simulink model "Quadrotor_Model_PID_Control_Updated"  (R2023b)
settings: Solver=VariableStepAuto  StartTime=0.0  StopTime=5  MaxStep=1e-2  RelTol=1e-3  AbsTol=1e-3
values from neighbouring files (symbols this model uses):
  b = 1.140 * 10^-7    (= 1.14e-07)    [Quadrotor_PID_Parameter_Trial_Updated.m]
  g = 9.82    [Quadrotor_PID_Parameter_Trial_Updated.m]
  I_xx = 4.856 * 10^-3    (= 0.004856)    [Quadrotor_PID_Parameter_Trial_Updated.m]
  I_yy = 4.856 * 10^-3    (= 0.004856)    [Quadrotor_PID_Parameter_Trial_Updated.m]
  I_zz = 8.801 * 10^-3    (= 0.008801)    [Quadrotor_PID_Parameter_Trial_Updated.m]
  k = 2.980*10^-6    (= 2.98e-06)    [Quadrotor_PID_Parameter_Trial_Updated.m]
  Kdphi = 0.25    [Quadrotor_PID_Parameter_Trial_Updated.m]
  Kdpsi = 0.25    [Quadrotor_PID_Parameter_Trial_Updated.m]
  Kdtheta = 0.25    [Quadrotor_PID_Parameter_Trial_Updated.m]
  Kdx = 0.25    [Quadrotor_PID_Parameter_Trial_Updated.m]
  Kdy = 0.25    [Quadrotor_PID_Parameter_Trial_Updated.m]
  Kdz = 0.25    [Quadrotor_PID_Parameter_Trial_Updated.m]
  Kiphi = 0.25    [Quadrotor_PID_Parameter_Trial_Updated.m]
  Kipsi = 0.25    [Quadrotor_PID_Parameter_Trial_Updated.m]
  Kitheta = 0.25    [Quadrotor_PID_Parameter_Trial_Updated.m]
  Kpphi = 2.5    [Quadrotor_PID_Parameter_Trial_Updated.m]
  Kpphi_attitude = 25    [Quadrotor_PID_Parameter_Trial_Updated.m]
  Kppsi = 2.5    [Quadrotor_PID_Parameter_Trial_Updated.m]
  Kppsi_attitude = 2.5    [Quadrotor_PID_Parameter_Trial_Updated.m]
  Kptheta = 2.5    [Quadrotor_PID_Parameter_Trial_Updated.m]
  Kptheta_attitude = 2.5    [Quadrotor_PID_Parameter_Trial_Updated.m]
  Kzd = 0.25    [Quadrotor_PID_Parameter_Trial_Updated.m]
  Kzi = 0.25    [Quadrotor_PID_Parameter_Trial_Updated.m]
  Kzp = 0.25    [Quadrotor_PID_Parameter_Trial_Updated.m]
  l = 0.225    [Quadrotor_PID_Parameter_Trial_Updated.m]    (also in Reference_Drone_Updated_PID.m = 0.15)
  m = 0.468    [Quadrotor_PID_Parameter_Trial_Updated.m]
  pitch_d = 0.01    [Quadrotor_PID_Parameter_Trial_Updated.m]
  roll_d = 0.01    [Quadrotor_PID_Parameter_Trial_Updated.m]
  yaw_d = 0.01    [Quadrotor_PID_Parameter_Trial_Updated.m]
  z_d = 1    [Quadrotor_PID_Parameter_Trial_Updated.m]
settings Model: Creator=jerss  LastModifiedBy=jerss

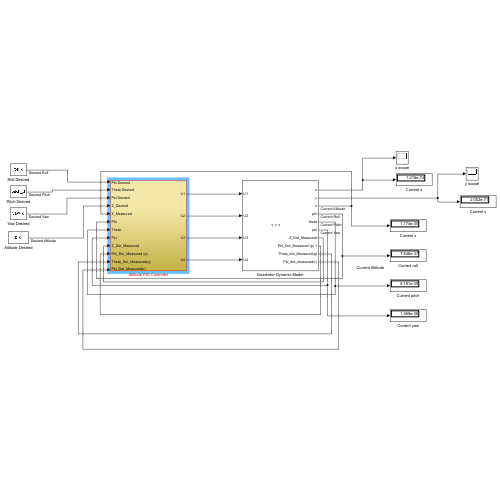
[thumbnail: Simulink's stored preview of the top-level diagram]
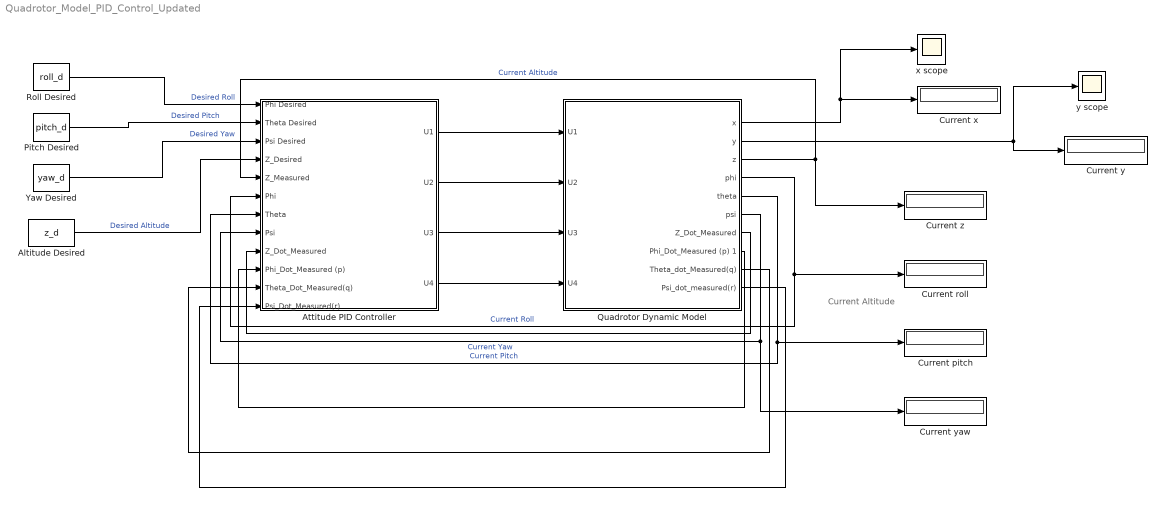
== system Quadrotor_Model_PID_Control_Updated ==
  note: Current Altitude
  Altitude Desired : Constant  Value=z_d
  Attitude PID Controller : Subsystem
  Current pitch : Display
  Current roll : Display
  Current x : Display
  Current y : Display
  Current yaw : Display
  Current z : Display
  Pitch Desired : Constant  Value=pitch_d
  Quadrotor Dynamic Model : Subsystem
      mask Display: image('C:\Users\angel\OneDrive - Universidad Politécnica de Yucatán\CIMAT\1st semester\Robotic Systems Modeling and Control\Project\Quadrotor\images\quadrotor.jpg');
  Roll Desired : Constant  Value=roll_d
  Yaw Desired : Constant  Value=yaw_d
  x scope : Scope
  y scope : Scope
  wires:
  Quadrotor Dynamic Model/3(z) -> Current z/1, Attitude PID Controller/5(Z_Measured)  "Current Altitude"
  Quadrotor Dynamic Model/4(phi) -> Current roll/1, Attitude PID Controller/6(Phi)  "Current Roll"
  Quadrotor Dynamic Model/5(theta) -> Current pitch/1, Attitude PID Controller/7(Theta)  "Current Pitch"
  Quadrotor Dynamic Model/6(psi) -> Current yaw/1, Attitude PID Controller/8(Psi)  "Current Yaw"
  Attitude PID Controller/1(U1) -> Quadrotor Dynamic Model/1(U1)
  Attitude PID Controller/2(U2) -> Quadrotor Dynamic Model/2(U2)
  Attitude PID Controller/3(U3) -> Quadrotor Dynamic Model/3(U3)
  Attitude PID Controller/4(U4) -> Quadrotor Dynamic Model/4(U4)
  Roll Desired/1 -> Attitude PID Controller/1(Phi Desired)  "Desired Roll"
  Pitch Desired/1 -> Attitude PID Controller/2(Theta Desired)  "Desired Pitch"
  Yaw Desired/1 -> Attitude PID Controller/3(Psi Desired)  "Desired Yaw"
  Altitude Desired/1 -> Attitude PID Controller/4(Z_Desired)  "Desired Altitude"
  Quadrotor Dynamic Model/1(x) -> x scope/1, Current x/1
  Quadrotor Dynamic Model/2(y) -> y scope/1, Current y/1
  Quadrotor Dynamic Model/7(Z_Dot_Measured) -> Attitude PID Controller/9(Z_Dot_Measured)
  Quadrotor Dynamic Model/8(Phi_Dot_Measured (p) 1) -> Attitude PID Controller/10(Phi_Dot_Measured (p))
  Quadrotor Dynamic Model/9(Theta_dot_Measured(q)) -> Attitude PID Controller/11(Theta_Dot_Measured(q))
  Quadrotor Dynamic Model/10(Psi_dot_measured(r)) -> Attitude PID Controller/12(Psi_Dot_Measured(r))

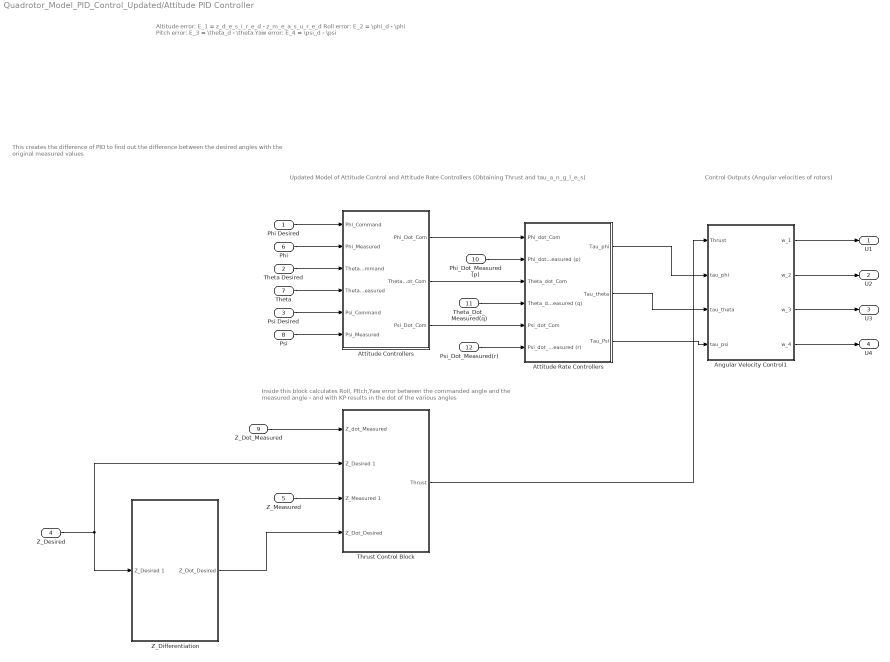
== system Quadrotor_Model_PID_Control_Updated/Attitude PID Controller ==
  note: Inside this block calculates Roll, PItch,Yaw error between the commanded angle and the measured angle - and with KP results in the dot of the various angles
  note: This creates the difference of PID to find out the difference between the desired angles with the original measured values
  note: Altitude error: E_1 = z_d_e_s_i_r_e_d - z_m_e_a_s_u_r_e_d
      | Roll error: E_2 = \phi_d - \phi
      | Pitch error: E_3 = \theta_d - \theta
      | Yaw error: E_4 = \psi_d - \psi
  note: Updated Model of Attitude Control and Attitude Rate Controllers
      | (Obtaining Thrust and tau_a_n_g_l_e_s)
  note: Control Outputs
      | (Angular velocities of rotors)
  Phi Desired : Inport
  Theta Desired : Inport  Port=2
  Psi Desired : Inport  Port=3
  Z_Desired : Inport  Port=4
  Z_Measured : Inport  Port=5
  Phi : Inport  Port=6
  Theta : Inport  Port=7
  Psi : Inport  Port=8
  Z_Dot_Measured : Inport  Port=9
  Phi_Dot_Measured (p) : Inport  Port=10
  Theta_Dot_Measured(q) : Inport  Port=11
  Psi_Dot_Measured(r) : Inport  Port=12
  Angular Velocity Control1 : Subsystem
  Attitude Controllers : Subsystem
  "Attitude Rate Controllers " : Subsystem
  Thrust Control Block : Subsystem
  Z_Differentiation : Subsystem
  U1 : Outport
  U2 : Outport  Port=2
  U3 : Outport  Port=3
  U4 : Outport  Port=4
  wires:
  Attitude Controllers/1(Phi_Dot_Com) -> "Attitude Rate Controllers "/1(Phi_dot_Com)
  Attitude Controllers/2(Theta_Dot_Com) -> "Attitude Rate Controllers "/3(Theta_dot_Com)
  Attitude Controllers/3(Psi_Dot_Com) -> "Attitude Rate Controllers "/5("Psi_dot_Com ")
  Angular Velocity Control1/4("w_4 ") -> U4/1
  Angular Velocity Control1/3(w_3) -> U3/1
  Angular Velocity Control1/2(w_2) -> U2/1
  Angular Velocity Control1/1(w_1) -> U1/1
  Thrust Control Block/1(Thrust) -> Angular Velocity Control1/1(Thrust)
  "Attitude Rate Controllers "/1(Tau_phi) -> Angular Velocity Control1/2(tau_phi)
  "Attitude Rate Controllers "/2(Tau_theta) -> Angular Velocity Control1/3(tau_theta)
  "Attitude Rate Controllers "/3(Tau_Psi) -> Angular Velocity Control1/4("tau_psi ")
  Z_Differentiation/1(Z_Dot_Desired) -> Thrust Control Block/4(Z_Dot_Desired)
  Phi Desired/1 -> Attitude Controllers/1(Phi_Command)
  Psi Desired/1 -> Attitude Controllers/5("Psi_Command ")
  Theta Desired/1 -> Attitude Controllers/3(Theta_Command)
  Phi/1 -> Attitude Controllers/2(Phi_Measured)
  Z_Desired/1 -> Thrust Control Block/2(Z_Desired 1), Z_Differentiation/1(Z_Desired 1)
  Z_Measured/1 -> Thrust Control Block/3(Z_Measured 1)
  Psi/1 -> Attitude Controllers/6("Psi_Measured ")
  Theta/1 -> Attitude Controllers/4(Theta_Measured)
  Z_Dot_Measured/1 -> Thrust Control Block/1(Z_dot_Measured)
  Phi_Dot_Measured (p)/1 -> "Attitude Rate Controllers "/2(Phi_dot_Measured (p))
  Theta_Dot_Measured(q)/1 -> "Attitude Rate Controllers "/4(Theta_dot_Measured (q))
  Psi_Dot_Measured(r)/1 -> "Attitude Rate Controllers "/6("Psi_dot_Measured (r) ")

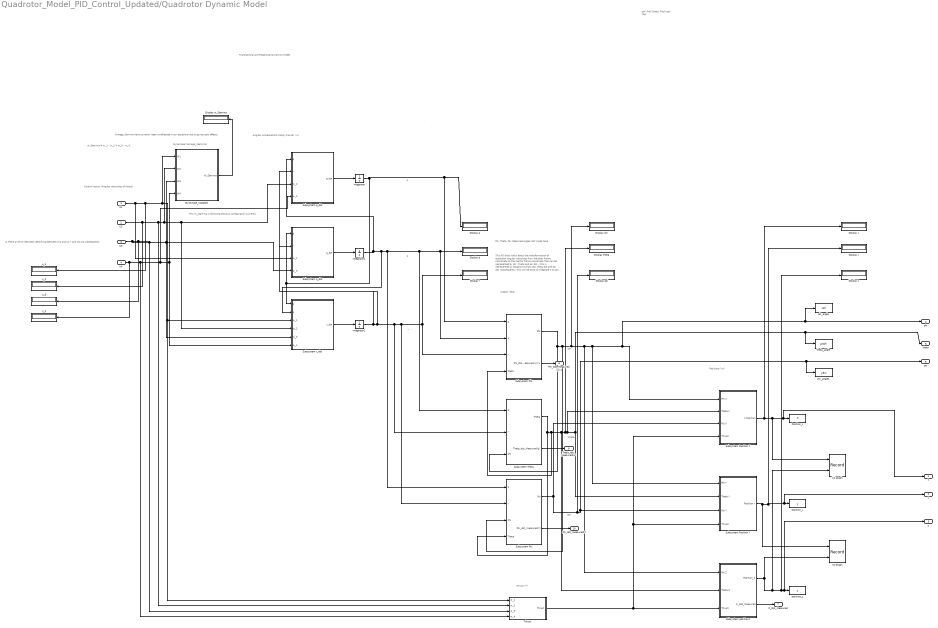
== system Quadrotor_Model_PID_Control_Updated/Quadrotor Dynamic Model ==
  note: w_Gamma = w_1 - w_2 + w_3 - w_4;
  note: Is there an error between identifying between W1 and U1 ? and W2,U2 subsequently
  note: Phi, Theta, Psi Measured angles dot inside here
  note: This W_Gamma is following the plus configuration currently
  note: Omega_Gamma have currently been unreflected in our equations due to gyroscopic effects
  note: This full block talks about the trabsformation of quadrotor angular velocities from the body frame coordinate to the inertial frame coordinate that can be represented by phi , theta and psi dot - this is represented by equation 6 of phi dot, theta dot and psi dot.
      | Subsequently, this will be done to integrate it to phi, theta and psi.
  note: Angular Accelerations (Body Frame) (\nu)
  note: .
  note: \phi: Roll
      | \theta: Pitch
      | \psi: Yaw
  note: Control Inputs
      | (Angular velocities of rotors)
  note: Positions (\xi)
  note: Angles (\eta)
  note: Gyroscope (\omega_\Gamma)
  note: Thrust (T)
  note: p
  note: q
  note: r
  note: \phi
  note: \theta
  note: \psi
  note: Translational and Rotational Dynamics Model
  U1 : Inport
  U2 : Inport  Port=2
  U3 : Inport  Port=3
  U4 : Inport  Port=4
  Display p : Display
  Display phi : Display
  Display psi : Display
  Display q : Display
  Display r : Display
  Display theta : Display
  Display w_Gamma : Display
  Display x : Display
  Display y : Display
  Display z : Display
  Gyroscope_Updated : Subsystem
  Integrator : Integrator
  Integrator1 : Integrator
  Integrator2 : Integrator
  Position_x : ToWorkspace  VariableName=X  SampleTime=-1
  Subsystem Phi : Subsystem
  Subsystem Position X : Subsystem
  Subsystem Position Y : Subsystem
  Subsystem Psi : Subsystem
  Subsystem Theta : Subsystem
  Subsystem p_dot : Subsystem
  Subsystem position z : Subsystem
  Subsystem q_dot : Subsystem
  Subsystem r_dot : Subsystem
  Thrust : MATLAB Function  TreatAsAtomicUnit=on
  XZ graph : Record  FileSettingsInternal="{\"entries\":[{\"content\":{\"excelSettings\":{\"content\":{},\"type\":\"Streamout.ExcelSettings\"}},\"type\":\"Streamout.FileSettingStorage\",\"uuid\":\"\"}],\"packageUris\":[\"http:\\/\\/schema.mathworks.com\\/mf0\\/streamout_blocks\\/R2020a\"],\"version\":\"1.0\"}"  Layout=[1 1]  SignalsInternal="{\"entries\":[{\"content\":{\"signals\":[{\"content\":{\"blockPath\":[],\"dimensions\":[1],\"domain\":\"\",\"lineColor\":\"#a2142f\",\"plots\":[1],\"port\":1,\"sid\":[\"\"],\"signalID\":59066,\"signalName\":\"Subsystem Position X\"},\"type\":\"RecordBlkView.Signal\",\"uuid\":\"\"},{\"content\":{\"blockPath\":[],\"dimensions\":[1],\"domain\":\"\",\"lineColor\":\"#139fff\",\"plots\":[1],\"port\":2,\"sid\":[\"\"],\"signalID\":59070,\"signalName\":\"Subsystem position z:1\"},\"type\":\"RecordBlkView.Signal\",\"uuid\":\"\"}]},\"type\":\"RecordBlkView.InputSignals\",\"uuid\":\"\"}],\"packageUris\":[\"http:\\/\\/schema.mathworks.com\\/mf0\\/streamout_blocks\\/R2020a\"],\"version\":\"1.0\"}"  VisualizationBindings="{\"xyplotplugin\":{\"info\":[{\"series\":[{\"bindingParametersList\":[{\"parameter\":\"X-Axis\",\"signalID\":59066,\"signalName\":\"Subsystem Position X\"},{\"parameter\":\"Y-Axis\",\"signalID\":59070,\"signalName\":\"Subsystem position z:1\"}],\"seriesID\":430}],\"subplotID\":1}]}}"  CompatibilityTag=XY  st=-1
  YZ Graph : Record  FileSettingsInternal="{\"entries\":[{\"content\":{\"excelSettings\":{\"content\":{},\"type\":\"Streamout.ExcelSettings\"}},\"type\":\"Streamout.FileSettingStorage\",\"uuid\":\"\"}],\"packageUris\":[\"http:\\/\\/schema.mathworks.com\\/mf0\\/streamout_blocks\\/R2020a\"],\"version\":\"1.0\"}"  Layout=[1 1]  SignalsInternal="{\"entries\":[{\"content\":{\"signals\":[{\"content\":{\"blockPath\":[],\"dimensions\":[1],\"domain\":\"\",\"lineColor\":\"#a2142f\",\"plots\":[1],\"port\":1,\"sid\":[\"\"],\"signalID\":59074,\"signalName\":\"Subsystem Position Y\"},\"type\":\"RecordBlkView.Signal\",\"uuid\":\"\"},{\"content\":{\"blockPath\":[],\"dimensions\":[1],\"domain\":\"\",\"lineColor\":\"#139fff\",\"plots\":[1],\"port\":2,\"sid\":[\"\"],\"signalID\":59078,\"signalName\":\"Subsystem position z:1\"},\"type\":\"RecordBlkView.Signal\",\"uuid\":\"\"}]},\"type\":\"RecordBlkView.InputSignals\",\"uuid\":\"\"}],\"packageUris\":[\"http:\\/\\/schema.mathworks.com\\/mf0\\/streamout_blocks\\/R2020a\"],\"version\":\"1.0\"}"  VisualizationBindings="{\"xyplotplugin\":{\"info\":[{\"series\":[{\"bindingParametersList\":[{\"parameter\":\"X-Axis\",\"signalID\":59074,\"signalName\":\"Subsystem Position Y\"},{\"parameter\":\"Y-Axis\",\"signalID\":59078,\"signalName\":\"Subsystem position z:1\"}],\"seriesID\":13612}],\"subplotID\":1}]}}"  CompatibilityTag=XY  st=-1
  phi_angle : ToWorkspace  VariableName=roll  SampleTime=-1
  phi_angle1 : ToWorkspace  VariableName=yaw  SampleTime=-1
  position_y : ToWorkspace  VariableName=y  SampleTime=-1
  position_z : ToWorkspace  VariableName=z  SampleTime=-1
  theta_angle : ToWorkspace  VariableName=pitch  SampleTime=-1
  u_{1..4} (4 alike) : Display
  x : Outport
  y : Outport  Port=2
  z : Outport  Port=3
  phi : Outport  Port=4
  theta : Outport  Port=5
  psi : Outport  Port=6
  Z_Dot_Measured : Outport  Port=7
  Phi_Dot_Measured (p) 1 : Outport  Port=8
  Theta_dot_Measured(q) : Outport  Port=9
  Psi_dot_measured(r) : Outport  Port=10
  wires:
  U1/1 -> Subsystem q_dot/3(w_1), u_1/1, Gyroscope_Updated/1(W1), Subsystem r_dot/3(w_1), Thrust/1(w_1)
  U2/1 -> Gyroscope_Updated/2(W2), Subsystem p_dot/3(w_2), Subsystem r_dot/4(w_2), Thrust/2(w_2), u_2/1
  U3/1 -> Subsystem q_dot/4(w_3), Gyroscope_Updated/3(W3), Subsystem r_dot/5(w_3), Thrust/3(w_3), u_3/1
  U4/1 -> u_4/1, Gyroscope_Updated/4(W4), Subsystem r_dot/6(w_4), Subsystem p_dot/4(w_4), Thrust/4(w_4)
  Thrust/1(Thrust) -> Subsystem Position X/4(Thrust), Subsystem Position Y/4("Thrust "), Subsystem position z/3(Thrust)
  Subsystem Phi/1("Phi ") -> Subsystem Theta/3("phi "), Subsystem Psi/3(Phi), Display phi/1, Subsystem position z/1("Phi Z "), Subsystem Position Y/1("Phi Y "), phi/1, phi_angle/1, Subsystem Position X/1("Phi X ")
  Subsystem Psi/1(Psi) -> Display psi/1, phi_angle1/1, psi/1, Subsystem Position Y/3("Psi Y "), Subsystem Position X/3("Psi X ")
  Subsystem Position X/1(X Position) -> Display x/1, x/1, Position_x/1, XZ graph/1
  Subsystem position z/1(Position_Z) -> XZ graph/2, z/1, position_z/1, Display z/1, YZ Graph/2
  Subsystem Position Y/1("Position Y ") -> y/1, position_y/1, Display y/1, YZ Graph/1
  Gyroscope_Updated/1(W_Gamma) -> Display w_Gamma/1
  Subsystem p_dot/1(p_dot) -> Integrator/1
  Subsystem q_dot/1(q_dot) -> Integrator1/1
  Subsystem r_dot/1(r_dot) -> Integrator2/1
  Integrator/1 -> Display p/1, Subsystem Phi/1(p), Subsystem r_dot/1("p "), Subsystem q_dot/1("p ")
  Integrator2/1 -> Subsystem Theta/2(r), Subsystem Psi/2(r), Display r/1, Subsystem Phi/3(r), Subsystem p_dot/2(r), Subsystem q_dot/2(r)
  Integrator1/1 -> Subsystem p_dot/1(q), Subsystem Psi/1(q), Subsystem Theta/1(q), Display q/1, Subsystem Phi/2(q), Subsystem r_dot/2(q)
  Subsystem Theta/1(Theta) -> Subsystem Psi/4(Theta), Subsystem Phi/4(theta), Subsystem position z/2("Theta Z "), Display theta/1, Subsystem Position X/2("Theta X "), theta_angle/1, theta/1, Subsystem Position Y/2("Theta Y ")
  Subsystem position z/2(Z_Dot_Measured) -> Z_Dot_Measured/1
  Subsystem Phi/2(Phi_Dot_Measured (p) 1) -> Phi_Dot_Measured (p) 1/1
  Subsystem Theta/2(Theta_dot_Measured(q)) -> Theta_dot_Measured(q)/1
  Subsystem Psi/2(Psi_dot_measured(r)) -> Psi_dot_measured(r)/1

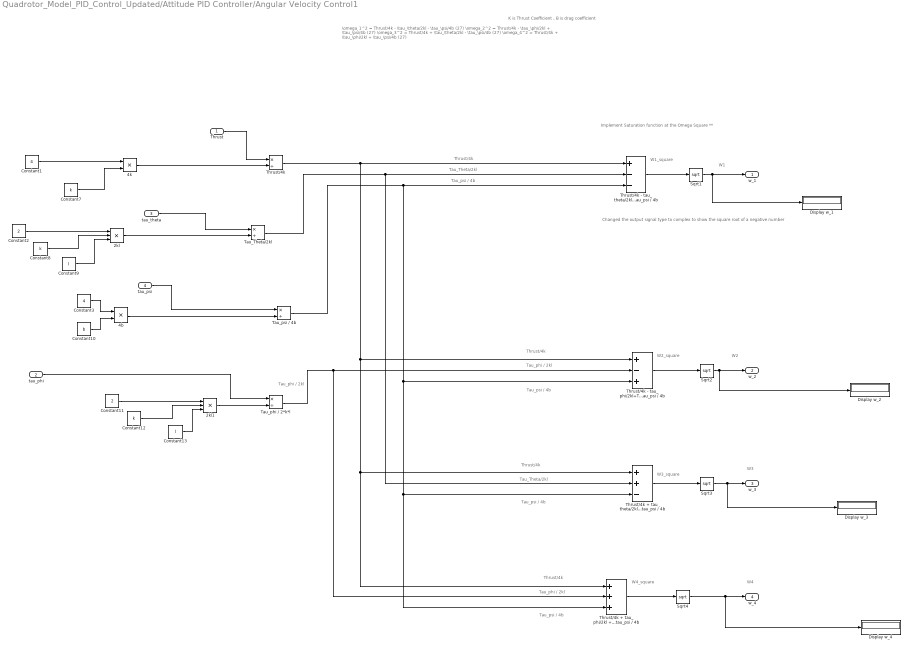
== system Quadrotor_Model_PID_Control_Updated/Attitude PID Controller/Angular Velocity Control1 ==
  note: Implement Saturation function at the Omega Square **
  note: Changed the output signal type to complex to show the square root of a negative number
  note: Tau_psi / 4b
  note: Tau_Theta/2kl
  note: Thrust/4k
  note: W1_square
  note: K is Thrust Coefficient , B is drag coefficient
  note: \omega_1^2 = Thrust/4k - \tau_\theta/2kl - \tau_\psi/4b   (27)
      |
      | \omega_2^2 = Thrust/4k - \tau_\phi/2kl + \tau_\psi/4b   (27)
      |
      | \omega_3^2 = Thrust/4k + \tau_\theta/2kl - \tau_\psi/4b   (27)
      |
      | \omega_4^2 = Thrust/4k + \tau_\phi/2kl + \tau_\psi/4b   (27)
  note: W1
  note: Thrust/4k
  note: Tau_phi / 2kl
  note: Tau_psi / 4b
  note: W2_square
  note: W2
  note: Thrust/4k
  note: W3
  note: W3_square
  note: Tau_Theta/2kl
  note: Tau_psi / 4b
  note: W4_square
  note: W4
  note: Thrust/4k
  note: Tau_phi / 2kl
  note: Tau_phi / 2kl
  note: Tau_psi / 4b
  Thrust : Inport
  tau_phi : Inport  Port=2
  tau_theta : Inport  Port=3
  "tau_psi " : Inport  Port=4
  2kl : Product  Inputs=***
  2kl1 : Product  Inputs=***
  4b : Product  Inputs=**
  4k : Product  Inputs=**
  Constant1 : Constant  Value=4
  Constant10 : Constant  Value=b
  Constant11 : Constant  Value=2
  Constant12 : Constant  Value=k
  Constant13 : Constant  Value=l
  Constant2 : Constant  Value=2
  Constant3 : Constant  Value=4
  Constant7 : Constant  Value=k
  Constant8 : Constant  Value=k
  Constant9 : Constant  Value=l
  Display w_{1..4} (4 alike) : Display
  Sqrt1 : Sqrt
  Sqrt2 : Sqrt  OutputSignalType=real
  Sqrt3 : Sqrt
  Sqrt4 : Sqrt
  Tau_Theta/2kl : Product  Inputs=*/
  Tau_phi / 2*k*l : Product  Inputs=*/
  Tau_psi / 4b : Product  Inputs=*/
  Thrust/4k : Product  Inputs=*/
  Thrust/4k + tau_phi/2kl + tau_psi / 4b : Sum  Inputs=+++
  Thrust/4k + tau_theta/2kl -tau_psi / 4b : Sum  Inputs=++-
  Thrust/4k - tau_phi/2kl+Tau_psi / 4b : Sum  Inputs=+-+
  Thrust/4k - tau_theta/2kl-Tau_psi / 4b : Sum  Inputs=+--
  w_1 : Outport
  w_2 : Outport  Port=2
  w_3 : Outport  Port=3
  "w_4 " : Outport  Port=4
  wires:
  tau_theta/1 -> Tau_Theta/2kl/1
  Sqrt1/1 -> Display w_1/1, w_1/1
  tau_phi/1 -> Tau_phi / 2*k*l/1
  "tau_psi "/1 -> Tau_psi / 4b/1
  Sqrt2/1 -> Display w_2/1, w_2/1
  Thrust/4k - tau_phi/2kl+Tau_psi / 4b/1 -> Sqrt2/1
  Thrust/4k + tau_theta/2kl -tau_psi / 4b/1 -> Sqrt3/1
  Sqrt3/1 -> Display w_3/1, w_3/1
  Thrust/4k + tau_phi/2kl + tau_psi / 4b/1 -> Sqrt4/1
  Sqrt4/1 -> Display w_4/1, "w_4 "/1
  Constant1/1 -> 4k/1
  Constant7/1 -> 4k/2
  Constant8/1 -> 2kl/2
  Constant2/1 -> 2kl/1
  2kl/1 -> Tau_Theta/2kl/2
  Constant9/1 -> 2kl/3
  Constant3/1 -> 4b/1
  Constant10/1 -> 4b/2
  4k/1 -> Thrust/4k/2
  Constant11/1 -> 2kl1/1
  Constant12/1 -> 2kl1/2
  Constant13/1 -> 2kl1/3
  Thrust/1 -> Thrust/4k/1
  4b/1 -> Tau_psi / 4b/2
  2kl1/1 -> Tau_phi / 2*k*l/2
  Thrust/4k/1 -> Thrust/4k + tau_theta/2kl -tau_psi / 4b/1, Thrust/4k + tau_phi/2kl + tau_psi / 4b/1, Thrust/4k - tau_phi/2kl+Tau_psi / 4b/1, Thrust/4k - tau_theta/2kl-Tau_psi / 4b/1
  Tau_Theta/2kl/1 -> Thrust/4k - tau_theta/2kl-Tau_psi / 4b/2, Thrust/4k + tau_theta/2kl -tau_psi / 4b/2
  Thrust/4k - tau_theta/2kl-Tau_psi / 4b/1 -> Sqrt1/1
  Tau_phi / 2*k*l/1 -> Thrust/4k + tau_phi/2kl + tau_psi / 4b/2, Thrust/4k - tau_phi/2kl+Tau_psi / 4b/2
  Tau_psi / 4b/1 -> Thrust/4k - tau_theta/2kl-Tau_psi / 4b/3, Thrust/4k - tau_phi/2kl+Tau_psi / 4b/3, Thrust/4k + tau_phi/2kl + tau_psi / 4b/3, Thrust/4k + tau_theta/2kl -tau_psi / 4b/3

== system Quadrotor_Model_PID_Control_Updated/Attitude PID Controller/Attitude Controllers ==
  note: Phi,Theta, Psi dot measured can be taken from the UAV Quadrotor Modelling
  note: Taken from Iris + Quadrotor Equations - on Attitude Controllers - Equation 57,58,59 - Can also follow 49.50.51.52.53 Eqn
  note: Yaw Rate Command
  note: Pitch Rate Command
  note: Roll Rate Command
  note: Utilising PD to minimise error in Z-Axis
      | Total Thrust T which affects the acceleration in the z- direction is set to equal to mg.
      | Constraint is enforced to keep the quadcopter flying.
      | Converting thrust equation to appropriate reference frame and utisiling PD to minimise the error in the Z-Axis
      |
      | T = (g + K_{z,D}(z_d_e_s_i_r_e_ddot - z_d_o_t) + K_{z,P}(z_d_e_s_i_r_e_d - z)) m/(C_\phiC_\theta)     (25)
      |
      | \tau_\phi = (K_{\phi,D}(\phi_d - \phi) + K_{\phi,P}(\phi_d - \phi)) I_{xx}                   (24)
      |
      | \tau_\theta = (K_{\theta,D}(\theta_d - \theta) + K_{\theta,P}(\theta_d - \theta)) I_{yy}                    (24)
      |
      | \tau_\psi = (K_{\psi,D}(\psi_d - \psi) + K_{\psi,P}(\psi_d - \psi)) I_{zz}                (24)
  Phi_Command : Inport
  Phi_Measured : Inport  Port=2
  Theta_Command : Inport  Port=3
  Theta_Measured : Inport  Port=4
  "Psi_Command " : Inport  Port=5
  "Psi_Measured " : Inport  Port=6
  Pitch error : Display
  Proportional Gain : Gain  Gain=Kpphi_attitude
  Proportional Gain1 : Gain  Gain=Kptheta_attitude
  Proportional Gain2 : Gain  Gain=Kppsi_attitude
  Roll error : Display
  Sum1 : Sum  Inputs=|+-
  Sum2 : Sum  Inputs=|+-
  Sum3 : Sum  Inputs=|+-
  Yaw error : Display
  Phi_Dot_Com : Outport
  Theta_Dot_Com : Outport  Port=2
  Psi_Dot_Com : Outport  Port=3
  wires:
  Phi_Command/1 -> Sum3/1
  Phi_Measured/1 -> Sum3/2
  Sum3/1 -> Roll error/1, Proportional Gain/1  "Roll Error"
  Theta_Command/1 -> Sum2/1
  Theta_Measured/1 -> Sum2/2
  Sum2/1 -> Pitch error/1, Proportional Gain1/1  "Pitch Error"
  "Psi_Command "/1 -> Sum1/1
  "Psi_Measured "/1 -> Sum1/2
  Sum1/1 -> Yaw error/1, Proportional Gain2/1  "Yaw Error"
  Proportional Gain/1 -> Phi_Dot_Com/1
  Proportional Gain1/1 -> Theta_Dot_Com/1
  Proportional Gain2/1 -> Psi_Dot_Com/1

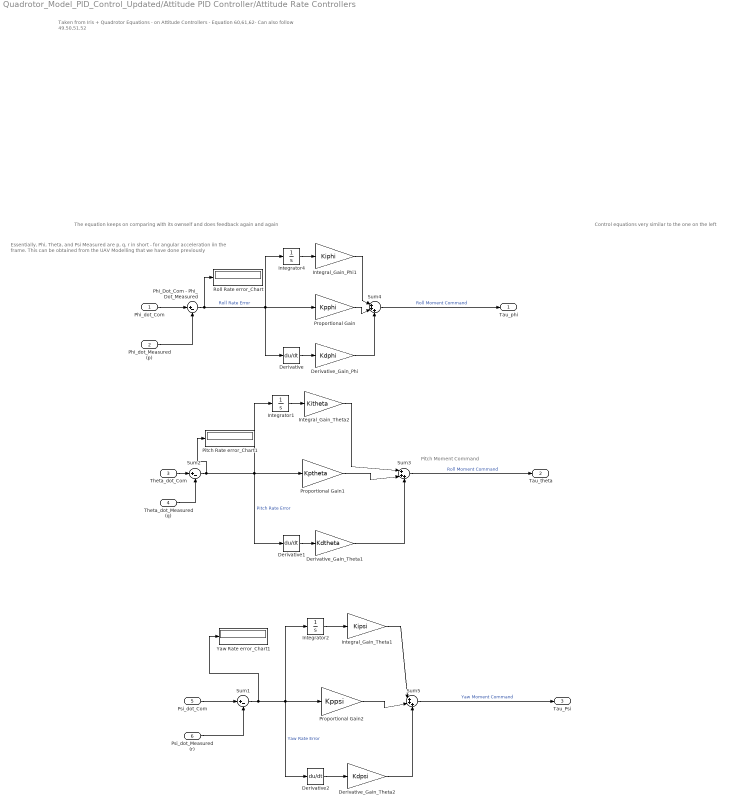
== system Quadrotor_Model_PID_Control_Updated/Attitude PID Controller/Attitude Rate Controllers  ==
  note: Essentially, Phi, Theta, and Psi Measured are p, q, r in short - for angular acceleration iin the frame. This can be obtained from the UAV Modelling that we have done previously
  note: Control equations very similar to the one on the left
  note: The equation keeps on comparing with its ownself and does feedback again and again
  note: Taken from Iris + Quadrotor Equations - on Attitude Controllers - Equation 60,61,62- Can also follow 49.50,51.52
  note: Pitch Moment Command
  Phi_dot_Com : Inport
  Phi_dot_Measured (p) : Inport  Port=2
  Theta_dot_Com : Inport  Port=3
  Theta_dot_Measured (q) : Inport  Port=4
  "Psi_dot_Com " : Inport  Port=5
  "Psi_dot_Measured (r) " : Inport  Port=6
  Derivative : Derivative
  Derivative1 : Derivative
  Derivative2 : Derivative
  Derivative_Gain_Phi : Gain  Gain=Kdphi
  Derivative_Gain_Theta1 : Gain  Gain=Kdtheta
  Derivative_Gain_Theta2 : Gain  Gain=Kdpsi
  Integral_Gain_Phi1 : Gain  Gain=Kiphi
  Integral_Gain_Theta1 : Gain  Gain=Kipsi
  Integral_Gain_Theta2 : Gain  Gain=Kitheta
  Integrator1 : Integrator
  Integrator2 : Integrator
  Integrator4 : Integrator
  Phi_Dot_Com - Phi_Dot_Measured : Sum  Inputs=|+-
  Pitch Rate error_Chart1 : Display
  Proportional Gain : Gain  Gain=Kpphi
  Proportional Gain1 : Gain  Gain=Kptheta
  Proportional Gain2 : Gain  Gain=Kppsi
  Roll Rate error_Chart : Display
  Sum1 : Sum  Inputs=|+-
  Sum2 : Sum  Inputs=|+-
  Sum3 : Sum  Inputs=|+++
  Sum4 : Sum  Inputs=|+++
  Sum5 : Sum  Inputs=|+++
  Yaw Rate error_Chart1 : Display
  Tau_phi : Outport
  Tau_theta : Outport  Port=2
  Tau_Psi : Outport  Port=3
  wires:
  Phi_dot_Com/1 -> Phi_Dot_Com - Phi_Dot_Measured/1
  Phi_dot_Measured (p)/1 -> Phi_Dot_Com - Phi_Dot_Measured/2
  Phi_Dot_Com - Phi_Dot_Measured/1 -> Roll Rate error_Chart/1, Integrator4/1, Derivative/1, Proportional Gain/1  "Roll Rate Error"
  Theta_dot_Com/1 -> Sum2/1
  Theta_dot_Measured (q)/1 -> Sum2/2
  Sum2/1 -> Pitch Rate error_Chart1/1, Derivative1/1, Integrator1/1, Proportional Gain1/1  "Pitch Rate Error"
  "Psi_dot_Com "/1 -> Sum1/1
  "Psi_dot_Measured (r) "/1 -> Sum1/2
  Sum1/1 -> Yaw Rate error_Chart1/1, Derivative2/1, Integrator2/1, Proportional Gain2/1  "Yaw Rate Error"
  Sum4/1 -> Tau_phi/1  "Roll Moment Command"
  Derivative/1 -> Derivative_Gain_Phi/1
  Integral_Gain_Phi1/1 -> Sum4/1
  Proportional Gain/1 -> Sum4/2
  Derivative_Gain_Phi/1 -> Sum4/3
  Integrator4/1 -> Integral_Gain_Phi1/1
  Integral_Gain_Theta2/1 -> Sum3/1
  Integrator1/1 -> Integral_Gain_Theta2/1
  Proportional Gain1/1 -> Sum3/2
  Derivative1/1 -> Derivative_Gain_Theta1/1
  Derivative_Gain_Theta1/1 -> Sum3/3
  Sum3/1 -> Tau_theta/1  "Roll Moment Command"
  Integral_Gain_Theta1/1 -> Sum5/1
  Integrator2/1 -> Integral_Gain_Theta1/1
  Sum5/1 -> Tau_Psi/1  "Yaw Moment Command"
  Proportional Gain2/1 -> Sum5/2
  Derivative2/1 -> Derivative_Gain_Theta2/1
  Derivative_Gain_Theta2/1 -> Sum5/3

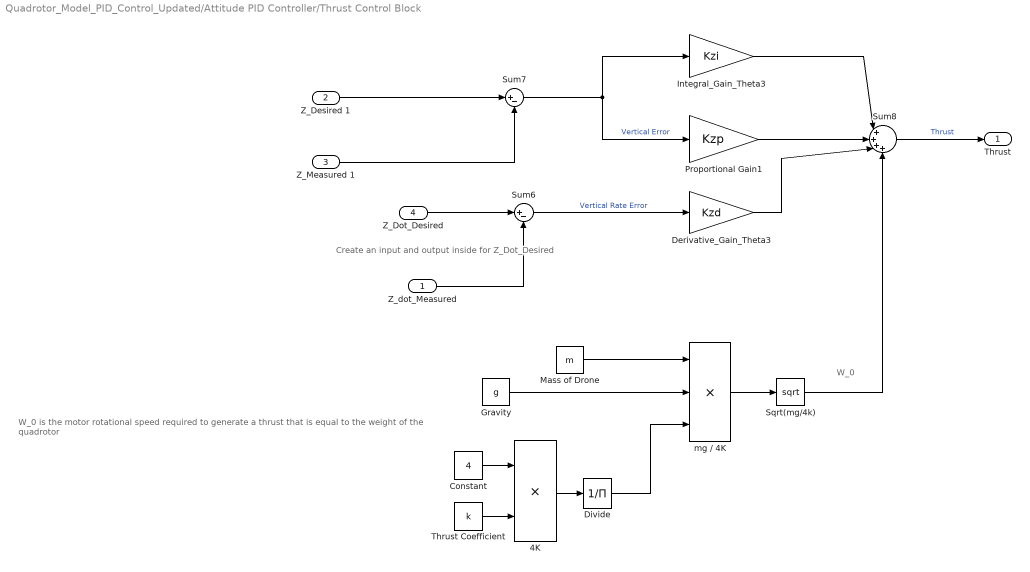
== system Quadrotor_Model_PID_Control_Updated/Attitude PID Controller/Thrust Control Block ==
  note: Create an input and output inside for Z_Dot_Desired
  note: W_0
  note: W_0 is the motor rotational speed required to generate a thrust that is equal to the weight of the quadrotor
  Z_dot_Measured : Inport
  Z_Desired 1 : Inport  Port=2
  Z_Measured 1 : Inport  Port=3
  Z_Dot_Desired : Inport  Port=4
  4K : Product
  Constant : Constant  Value=4
  Derivative_Gain_Theta3 : Gain  Gain=Kzd
  Divide : Product  Inputs=/
  Gravity : Constant  Value=g
  Integral_Gain_Theta3 : Gain  Gain=Kzi
  Mass of Drone : Constant  Value=m
  Proportional Gain1 : Gain  Gain=Kzp
  Sqrt(mg/4k) : Sqrt
  Sum6 : Sum  Inputs=|+-
  Sum7 : Sum  Inputs=|+-
  Sum8 : Sum  Inputs=|++++
  Thrust Coefficient : Constant  Value=k
  mg / 4K : Product  Inputs=3
  Thrust : Outport
  wires:
  Sqrt(mg/4k)/1 -> Sum8/4
  Sum8/1 -> Thrust/1  "Thrust"
  Integral_Gain_Theta3/1 -> Sum8/1
  Z_dot_Measured/1 -> Sum6/2
  mg / 4K/1 -> Sqrt(mg/4k)/1
  Gravity/1 -> mg / 4K/2
  Divide/1 -> mg / 4K/3
  4K/1 -> Divide/1
  Mass of Drone/1 -> mg / 4K/1
  Constant/1 -> 4K/1
  Z_Desired 1/1 -> Sum7/1
  Derivative_Gain_Theta3/1 -> Sum8/3
  Proportional Gain1/1 -> Sum8/2
  Z_Dot_Desired/1 -> Sum6/1
  Thrust Coefficient/1 -> 4K/2
  Sum7/1 -> Proportional Gain1/1, Integral_Gain_Theta3/1  "Vertical Error"
  Sum6/1 -> Derivative_Gain_Theta3/1  "Vertical Rate Error"
  Z_Measured 1/1 -> Sum7/2

== system Quadrotor_Model_PID_Control_Updated/Attitude PID Controller/Z_Differentiation ==
  Z_Desired 1 : Inport
  Derivative : Derivative
  Z_Dot_Desired : Outport
  wires:
  Z_Desired 1/1 -> Derivative/1
  Derivative/1 -> Z_Dot_Desired/1

== system Quadrotor_Model_PID_Control_Updated/Quadrotor Dynamic Model/Gyroscope_Updated ==
  note: w_Gamma = w_1 - w_2 + w_3 - w_4;
  W1 : Inport
  W2 : Inport  Port=2
  W3 : Inport  Port=3
  W4 : Inport  Port=4
  W1-W2+W3-W4 : Sum  Inputs=+-+-
  W_Gamma : Outport
  wires:
  W1/1 -> W1-W2+W3-W4/1
  W2/1 -> W1-W2+W3-W4/2
  W3/1 -> W1-W2+W3-W4/3
  W4/1 -> W1-W2+W3-W4/4
  W1-W2+W3-W4/1 -> W_Gamma/1

== system Quadrotor_Model_PID_Control_Updated/Quadrotor Dynamic Model/Subsystem Phi ==
  note: Angular Velocity of Phi in the Inertial Frame = Wi
  note: \phi
  note: \phi
  note: .
  note: \phi = p + q(S_\phiT_\theta) + r(C_\phiT_\theta) (6)
  note: .
  note: Display for \phi
  p : Inport
  q : Inport  Port=2
  r : Inport  Port=3
  theta : Inport  Port=4
  "Cos_phi " : Trigonometry  Operator=cos
  Display for q*sin(phi)*tan(Theta) : Display
  Display1 : Display
  Display10 : Display
  Integrator6 : Integrator
  Tan Theta : Trigonometry  Operator=tan
  Tan_Theta : Trigonometry  Operator=tan
  p+ q (sphi ttheta) + r( cphi ttheta) : Sum  Inputs=+++
  q*sin(phi)*tan(Theta) : Product  Inputs=3
  r*cos(phi)*tan(theta) : Product  Inputs=3
  sin(phi) : Trigonometry
  "Phi " : Outport
  Phi_Dot_Measured (p) 1 : Outport  Port=2
  wires:
  "Cos_phi "/1 -> r*cos(phi)*tan(theta)/1
  r*cos(phi)*tan(theta)/1 -> Display10/1, p+ q (sphi ttheta) + r( cphi ttheta)/1
  theta/1 -> Tan_Theta/1, Tan Theta/1
  Integrator6/1 -> "Cos_phi "/1, Display1/1, sin(phi)/1, "Phi "/1
  Tan Theta/1 -> r*cos(phi)*tan(theta)/3
  p+ q (sphi ttheta) + r( cphi ttheta)/1 -> Phi_Dot_Measured (p) 1/1, Integrator6/1
  q/1 -> q*sin(phi)*tan(Theta)/2
  q*sin(phi)*tan(Theta)/1 -> Display for q*sin(phi)*tan(Theta)/1, p+ q (sphi ttheta) + r( cphi ttheta)/3
  p/1 -> p+ q (sphi ttheta) + r( cphi ttheta)/2
  sin(phi)/1 -> q*sin(phi)*tan(Theta)/1
  Tan_Theta/1 -> q*sin(phi)*tan(Theta)/3
  r/1 -> r*cos(phi)*tan(theta)/2

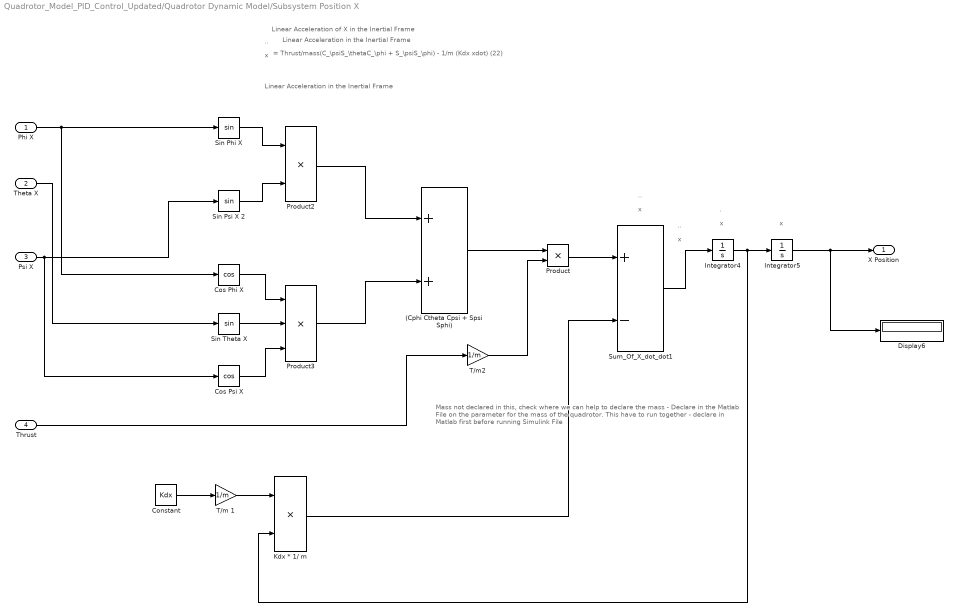
== system Quadrotor_Model_PID_Control_Updated/Quadrotor Dynamic Model/Subsystem Position X ==
  note: ..
  note: x
  note: .
  note: x
  note: = Thrust/mass(C_\psiS_\thetaC_\phi + S_\psiS_\phi) - 1/m (Kdx xdot) (22)
  note: ..
  note: x
  note: Linear Acceleration of X in the Inertial Frame
  note: x
  note: Linear Acceleration in the Inertial Frame
  note: Linear Acceleration in the Inertial Frame
  note: Mass not declared in this, check where we can help to declare the mass - Declare in the Matlab File on the parameter for the mass of the quadrotor. This have to run together - declare in Matlab first before running Simulink File
  note: x
  note: ..
  "Phi X " : Inport
  "Theta X " : Inport  Port=2
  "Psi X " : Inport  Port=3
  Thrust : Inport  Port=4
  (Cphi Ctheta Cpsi + Spsi Sphi) : Sum
  Constant : Constant  Value=Kdx
  Cos Phi X : Trigonometry  Operator=cos
  Cos Psi X : Trigonometry  Operator=cos
  Display6 : Display
  Integrator4 : Integrator
  Integrator5 : Integrator
  Kdx * 1/ m : Product
  Product : Product
  Product2 : Product
  Product3 : Product  Inputs=3
  Sin Phi X : Trigonometry
  Sin Psi X 2 : Trigonometry
  "Sin Theta X " : Trigonometry
  Sum_Of_X_dot_dot1 : Sum  Inputs=+-
  T/m 1 : Gain  Gain=1/m
  T/m2 : Gain  Gain=1/m
  X Position : Outport
  wires:
  "Phi X "/1 -> Cos Phi X/1, Sin Phi X/1
  "Psi X "/1 -> Sin Psi X 2/1, Cos Psi X/1
  Product2/1 -> (Cphi Ctheta Cpsi + Spsi Sphi)/1
  Product3/1 -> (Cphi Ctheta Cpsi + Spsi Sphi)/2
  "Theta X "/1 -> "Sin Theta X "/1
  Sin Phi X/1 -> Product2/1
  "Sin Theta X "/1 -> Product3/2
  Sin Psi X 2/1 -> Product2/2
  Cos Psi X/1 -> Product3/3
  Cos Phi X/1 -> Product3/1
  Integrator5/1 -> X Position/1, Display6/1
  T/m2/1 -> Product/2
  Thrust/1 -> T/m2/1
  (Cphi Ctheta Cpsi + Spsi Sphi)/1 -> Product/1
  T/m 1/1 -> Kdx * 1/ m/1
  Constant/1 -> T/m 1/1
  Integrator4/1 -> Kdx * 1/ m/2, Integrator5/1
  Product/1 -> Sum_Of_X_dot_dot1/1
  Kdx * 1/ m/1 -> Sum_Of_X_dot_dot1/2
  Sum_Of_X_dot_dot1/1 -> Integrator4/1

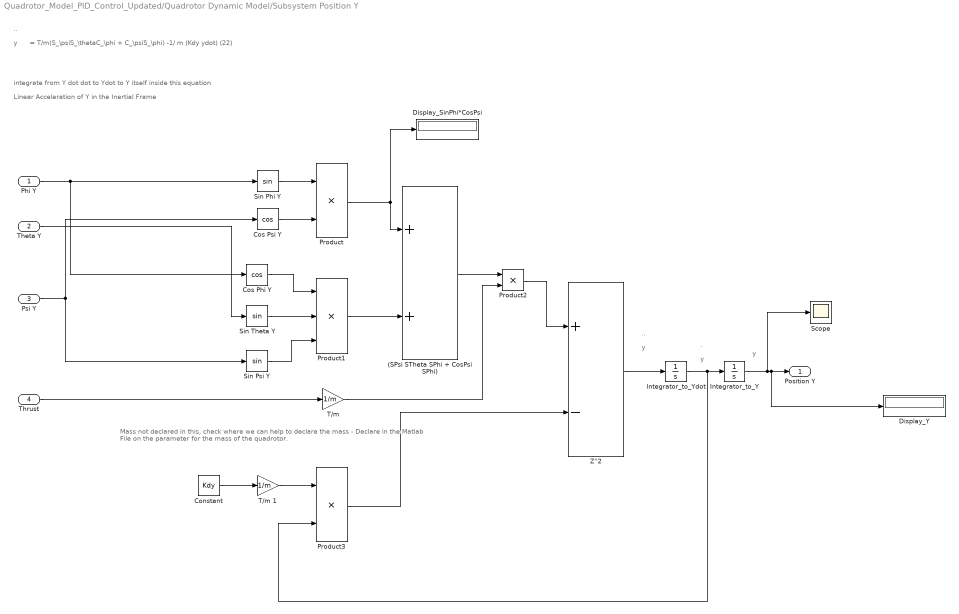
== system Quadrotor_Model_PID_Control_Updated/Quadrotor Dynamic Model/Subsystem Position Y ==
  note: Linear Acceleration of Y in the Inertial Frame
  note: integrate from Y dot dot to Ydot to Y itself inside this equation
  note: = T/m(S_\psiS_\thetaC_\phi + C_\psiS_\phi) -1/ m (Kdy ydot) (22)
  note: ..
  note: y
  note: y
  note: .
  note: ..
  note: y
  note: y
  note: Mass not declared in this, check where we can help to declare the mass - Declare in the Matlab File on the parameter for the mass of the quadrotor.
  "Phi Y " : Inport
  "Theta Y " : Inport  Port=2
  "Psi Y " : Inport  Port=3
  "Thrust " : Inport  Port=4
  " (SPsi STheta SPhi + CosPsi SPhi)" : Sum
  Constant : Constant  Value=Kdy
  Cos Phi Y : Trigonometry  Operator=cos
  Cos Psi Y : Trigonometry  Operator=cos
  Display_SinPhi*CosPsi : Display
  Display_Y : Display
  Integrator_to_Y : Integrator
  Integrator_to_Ydot : Integrator
  Product : Product
  Product1 : Product  Inputs=3
  Product2 : Product
  Product3 : Product
  Scope : Scope
  "Sin Phi Y " : Trigonometry
  Sin Psi Y : Trigonometry
  "Sin Theta Y " : Trigonometry
  "T/m " : Gain  Gain=1/m
  T/m 1 : Gain  Gain=1/m
  Z''2 : Sum  Inputs=+-
  "Position Y " : Outport
  wires:
  "Theta Y "/1 -> "Sin Theta Y "/1
  Integrator_to_Y/1 -> Display_Y/1, "Position Y "/1, Scope/1
  "Phi Y "/1 -> "Sin Phi Y "/1, Cos Phi Y/1
  Product/1 -> " (SPsi STheta SPhi + CosPsi SPhi)"/1, Display_SinPhi*CosPsi/1
  Cos Psi Y/1 -> Product/2
  "Psi Y "/1 -> Cos Psi Y/1, Sin Psi Y/1
  Sin Psi Y/1 -> Product1/3
  Product1/1 -> " (SPsi STheta SPhi + CosPsi SPhi)"/2
  Cos Phi Y/1 -> Product1/1
  "Sin Theta Y "/1 -> Product1/2
  "Sin Phi Y "/1 -> Product/1
  " (SPsi STheta SPhi + CosPsi SPhi)"/1 -> Product2/1
  "T/m "/1 -> Product2/2
  "Thrust "/1 -> "T/m "/1
  Integrator_to_Ydot/1 -> Integrator_to_Y/1, Product3/2
  Constant/1 -> T/m 1/1
  T/m 1/1 -> Product3/1
  Product2/1 -> Z''2/1
  Product3/1 -> Z''2/2
  Z''2/1 -> Integrator_to_Ydot/1

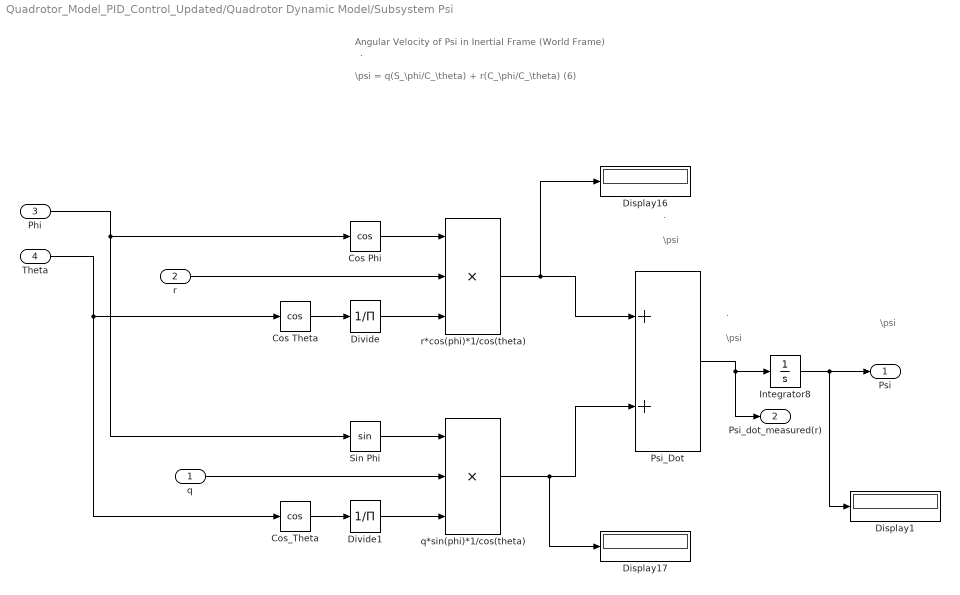
== system Quadrotor_Model_PID_Control_Updated/Quadrotor Dynamic Model/Subsystem Psi ==
  note: Angular Velocity of Psi in Inertial Frame (World Frame)
  note: .
  note: \psi
  note: \psi
  note: \psi = q(S_\phi/C_\theta) + r(C_\phi/C_\theta) (6)
  note: .
  note: \psi
  note: .
  q : Inport
  r : Inport  Port=2
  Phi : Inport  Port=3
  Theta : Inport  Port=4
  Cos Phi : Trigonometry  Operator=cos
  Cos Theta : Trigonometry  Operator=cos
  Cos_Theta : Trigonometry  Operator=cos
  Display1 : Display
  Display16 : Display
  Display17 : Display
  Divide : Product  Inputs=/
  Divide1 : Product  Inputs=/
  Integrator8 : Integrator
  Psi_Dot : Sum
  Sin Phi : Trigonometry
  q*sin(phi)*1/cos(theta) : Product  Inputs=3
  r*cos(phi)*1/cos(theta) : Product  Inputs=3
  Psi : Outport
  Psi_dot_measured(r) : Outport  Port=2
  wires:
  Cos Phi/1 -> r*cos(phi)*1/cos(theta)/1
  Divide1/1 -> q*sin(phi)*1/cos(theta)/3
  Sin Phi/1 -> q*sin(phi)*1/cos(theta)/1
  Cos Theta/1 -> Divide/1
  Divide/1 -> r*cos(phi)*1/cos(theta)/3
  Cos_Theta/1 -> Divide1/1
  r*cos(phi)*1/cos(theta)/1 -> Display16/1, Psi_Dot/1
  Theta/1 -> Cos_Theta/1, Cos Theta/1
  Phi/1 -> Sin Phi/1, Cos Phi/1
  q/1 -> q*sin(phi)*1/cos(theta)/2
  r/1 -> r*cos(phi)*1/cos(theta)/2
  Psi_Dot/1 -> Psi_dot_measured(r)/1, Integrator8/1
  q*sin(phi)*1/cos(theta)/1 -> Psi_Dot/2, Display17/1
  Integrator8/1 -> Display1/1, Psi/1

== system Quadrotor_Model_PID_Control_Updated/Quadrotor Dynamic Model/Subsystem Theta ==
  note: Initialise the Pitch Function for parameter initialisation
  note: Angular Velocity of Theta in Inertial Frame (World Frame)
  note: \theta
  note: .
  note: \theta
  note: .
  note: \theta = q(C_\phi) - r(S_\phi) (6)
  note: \theta
  note: .
  q : Inport
  r : Inport  Port=2
  "phi " : Inport  Port=3
  Cos Phi : Trigonometry  Operator=cos
  Display1 : Display
  Display13 : Display
  Display14 : Display
  Integrator_Thetadot to Theta : Integrator
  Sin_Phi : Trigonometry
  Z''4 : Sum  Inputs=-+
  q*cos(phi) : Product
  r*sin(phi) : Product
  Theta : Outport
  Theta_dot_Measured(q) : Outport  Port=2
  wires:
  "phi "/1 -> Cos Phi/1, Sin_Phi/1
  r/1 -> r*sin(phi)/2
  Cos Phi/1 -> q*cos(phi)/1
  q*cos(phi)/1 -> Display14/1, Z''4/2
  Z''4/1 -> Theta_dot_Measured(q)/1, Integrator_Thetadot to Theta/1
  Sin_Phi/1 -> r*sin(phi)/1
  r*sin(phi)/1 -> Display13/1, Z''4/1
  q/1 -> q*cos(phi)/2
  Integrator_Thetadot to Theta/1 -> Display1/1, Theta/1

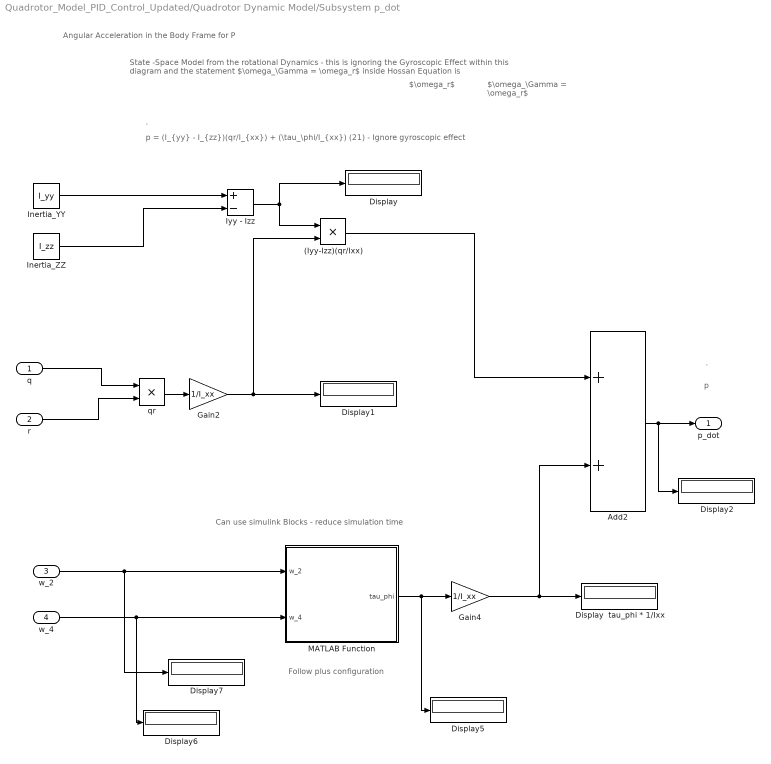
== system Quadrotor_Model_PID_Control_Updated/Quadrotor Dynamic Model/Subsystem p_dot ==
  note: Can use simulink Blocks - reduce simulation time
  note: .
  note: p
  note: Angular Acceleration in the Body Frame for P
  note: Follow plus configuration
  note: $\omega_r$
  note: $\omega_\Gamma = \omega_r$
  note: State -Space Model from the rotational Dynamics - this is ignoring the Gyroscopic Effect within this diagram and the statement $\omega_\Gamma = \omega_r$ inside Hossan Equation is
  note: p = (I_{yy} - I_{zz})(qr/I_{xx}) + (\tau_\phi/I_{xx}) (21) - Ignore gyroscopic effect
  note: .
  q : Inport
  r : Inport  Port=2
  w_2 : Inport  Port=3
  w_4 : Inport  Port=4
  (Iyy-Izz)(qr/Ixx) : Product
  Add2 : Sum
  Display{,1..2,5..7} (6 alike) : Display
  Display  tau_phi * 1/Ixx : Display
  Gain2 : Gain  Gain=1/I_xx
  Gain4 : Gain  Gain=1/I_xx
  Inertia_YY : Constant  Value=I_yy
  Inertia_ZZ : Constant  Value=I_zz
  Iyy - Izz : Sum  Inputs=+-
  MATLAB Function : MATLAB Function  TreatAsAtomicUnit=on
  qr : Product
  p_dot : Outport
  wires:
  Inertia_YY/1 -> Iyy - Izz/1
  Inertia_ZZ/1 -> Iyy - Izz/2
  Iyy - Izz/1 -> (Iyy-Izz)(qr/Ixx)/1, Display/1
  Add2/1 -> p_dot/1, Display2/1
  q/1 -> qr/1
  MATLAB Function/1(tau_phi) -> Display5/1, Gain4/1
  w_2/1 -> MATLAB Function/1(w_2), Display7/1
  w_4/1 -> Display6/1, MATLAB Function/2(w_4)
  Gain4/1 -> Display  tau_phi * 1/Ixx/1, Add2/2
  r/1 -> qr/2
  qr/1 -> Gain2/1
  Gain2/1 -> (Iyy-Izz)(qr/Ixx)/2, Display1/1
  (Iyy-Izz)(qr/Ixx)/1 -> Add2/1

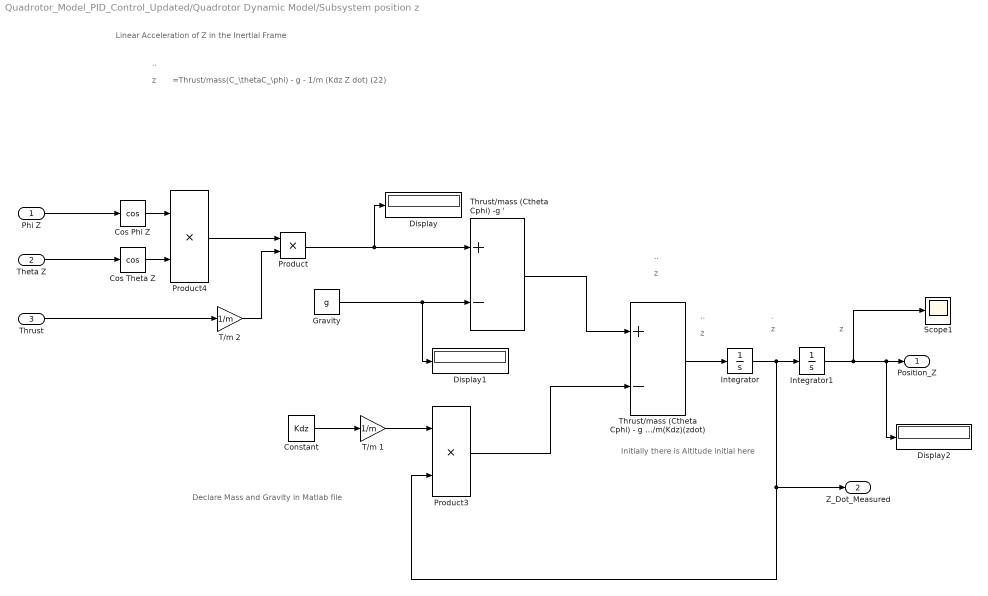
== system Quadrotor_Model_PID_Control_Updated/Quadrotor Dynamic Model/Subsystem position z ==
  note: Initially there is Altitude initial here
  note: Linear Acceleration of Z in the Inertial Frame
  note: Declare Mass and Gravity in Matlab file
  note: z
  note: ..
  note: .
  note: z
  note: =Thrust/mass(C_\thetaC_\phi) - g - 1/m (Kdz Z dot) (22)
  note: ..
  note: z
  note: z
  note: ..
  note: z
  "Phi Z " : Inport
  "Theta Z " : Inport  Port=2
  Thrust : Inport  Port=3
  Constant : Constant  Value=Kdz
  Cos Phi Z : Trigonometry  Operator=cos
  Cos Theta Z : Trigonometry  Operator=cos
  Display : Display
  Display1 : Display
  Display2 : Display
  Gravity : Constant  Value=g
  Integrator : Integrator
  Integrator1 : Integrator
  Product : Product
  Product3 : Product
  Product4 : Product
  Scope1 : Scope
  T/m 1 : Gain  Gain=1/m
  T/m 2 : Gain  Gain=1/m
  Thrust/mass (Ctheta Cphi) - g + - 1/m(Kdz)(zdot) : Sum  Inputs=+-
  Thrust/mass (Ctheta Cphi) -g ' : Sum  Inputs=+-
  Position_Z : Outport
  Z_Dot_Measured : Outport  Port=2
  wires:
  "Phi Z "/1 -> Cos Phi Z/1
  Gravity/1 -> Display1/1, Thrust/mass (Ctheta Cphi) -g '/2
  Integrator1/1 -> Position_Z/1, Display2/1, Scope1/1
  "Theta Z "/1 -> Cos Theta Z/1
  Integrator/1 -> Z_Dot_Measured/1, Product3/2, Integrator1/1
  Cos Theta Z/1 -> Product4/2
  Cos Phi Z/1 -> Product4/1
  Thrust/1 -> T/m 2/1
  Product4/1 -> Product/1
  Product/1 -> Display/1, Thrust/mass (Ctheta Cphi) -g '/1
  T/m 2/1 -> Product/2
  T/m 1/1 -> Product3/1
  Constant/1 -> T/m 1/1
  Thrust/mass (Ctheta Cphi) -g '/1 -> Thrust/mass (Ctheta Cphi) - g + - 1/m(Kdz)(zdot)/1
  Product3/1 -> Thrust/mass (Ctheta Cphi) - g + - 1/m(Kdz)(zdot)/2
  Thrust/mass (Ctheta Cphi) - g + - 1/m(Kdz)(zdot)/1 -> Integrator/1

== system Quadrotor_Model_PID_Control_Updated/Quadrotor Dynamic Model/Subsystem q_dot ==
  note: .
  note: q
  note: Angular Acceleration for Body Frame on Q
  note: This is on the Plus Configuration
  note: q = (I_{zz} - I_{xx})(pr/I_{yy}) + (\tau_\theta/I_{yy}) (11)
  note: .
  "p " : Inport
  r : Inport  Port=2
  w_1 : Inport  Port=3
  w_3 : Inport  Port=4
  Add3 : Sum
  Constant : Constant  Value=I_zz
  Constant1 : Constant  Value=I_xx
  Display{,1..2,4} (4 alike) : Display
  Gain2 : Gain  Gain=1/I_yy
  Gain5 : Gain  Gain=1/I_yy
  Izz - Ixx : Sum  Inputs=+-
  MATLAB Function1 : MATLAB Function  TreatAsAtomicUnit=on
  p*r(1/Iyy) : Product
  p*r(1/Iyy) * (Izz-Ixx) : Product
  q_dot : Outport
  wires:
  Constant/1 -> Izz - Ixx/1
  Constant1/1 -> Izz - Ixx/2
  Izz - Ixx/1 -> Display/1, p*r(1/Iyy) * (Izz-Ixx)/1
  p*r(1/Iyy)/1 -> p*r(1/Iyy) * (Izz-Ixx)/2, Display1/1
  r/1 -> Gain2/1
  Gain2/1 -> p*r(1/Iyy)/2
  "p "/1 -> p*r(1/Iyy)/1
  w_3/1 -> MATLAB Function1/2(w_3)
  MATLAB Function1/1(tau_theta) -> Gain5/1
  w_1/1 -> MATLAB Function1/1(w_1)
  Add3/1 -> q_dot/1, Display2/1
  Gain5/1 -> Display4/1, Add3/2
  p*r(1/Iyy) * (Izz-Ixx)/1 -> Add3/1

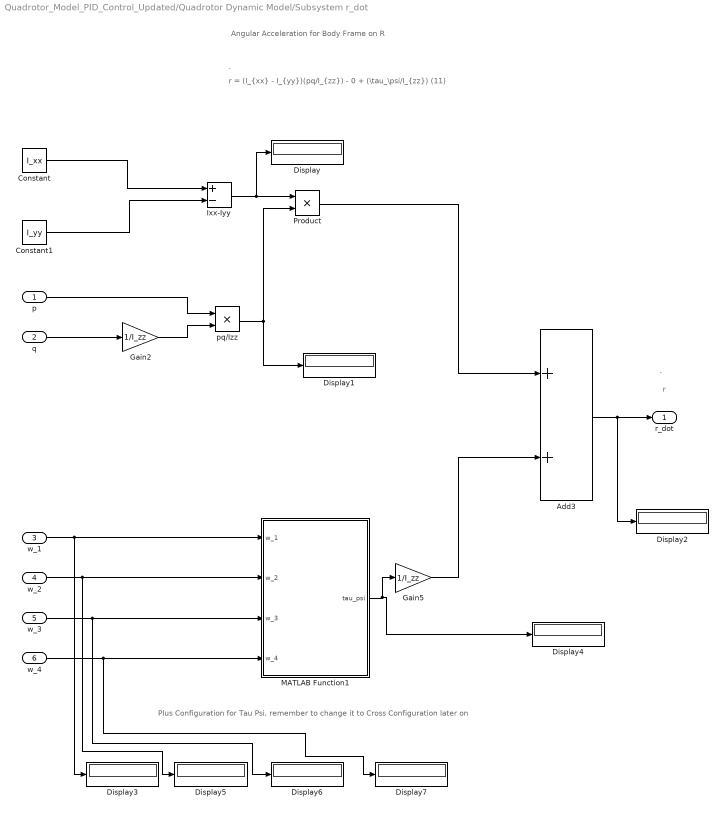
== system Quadrotor_Model_PID_Control_Updated/Quadrotor Dynamic Model/Subsystem r_dot ==
  note: r
  note: Plus Configuration for Tau Psi, remember to change it to Cross Configuration later on
  note: Angular Acceleration for Body Frame on R
  note: r = (I_{xx} - I_{yy})(pq/I_{zz}) - 0 + (\tau_\psi/I_{zz}) (11)
  note: .
  note: .
  "p " : Inport
  q : Inport  Port=2
  w_1 : Inport  Port=3
  w_2 : Inport  Port=4
  w_3 : Inport  Port=5
  w_4 : Inport  Port=6
  Add3 : Sum
  Constant : Constant  Value=I_xx
  Constant1 : Constant  Value=I_yy
  Display{,1..7} (8 alike) : Display
  Gain2 : Gain  Gain=1/I_zz
  Gain5 : Gain  Gain=1/I_zz
  Ixx-Iyy : Sum  Inputs=+-
  MATLAB Function1 : MATLAB Function  TreatAsAtomicUnit=on
  Product : Product
  pq/Izz : Product
  r_dot : Outport
  wires:
  Constant/1 -> Ixx-Iyy/1
  Constant1/1 -> Ixx-Iyy/2
  Ixx-Iyy/1 -> Display/1, Product/1
  pq/Izz/1 -> Display1/1, Product/2
  Add3/1 -> Display2/1, r_dot/1
  "p "/1 -> pq/Izz/1
  Gain2/1 -> pq/Izz/2
  q/1 -> Gain2/1
  MATLAB Function1/1(tau_psi) -> Display4/1, Gain5/1
  w_1/1 -> MATLAB Function1/1(w_1), Display3/1
  w_2/1 -> MATLAB Function1/2(w_2), Display5/1
  w_4/1 -> MATLAB Function1/4(w_4), Display7/1
  Gain5/1 -> Add3/2
  w_3/1 -> MATLAB Function1/3(w_3), Display6/1
  Product/1 -> Add3/1

== matlab function Quadrotor_Model_PID_Control_Updated/Quadrotor Dynamic Model/Subsystem r_dot/MATLAB Function1 ==
  data: w_1 input; w_2 input; w_3 input; tau_psi output; w_4 input
function tau_psi = fcn(w_1, w_2, w_3, w_4)
k = 2.980e-6; % Thrust factor of rotor (depends on density
              % geometry, etc) 
l = 0.225; % Linear distance from the centre of the rotor
           % to the centre of gravity    
b = 1.140e-7; % Drag constant
Im = 3.357e-5; % Inertia moment of the rotor
tau_psi = b*(-w_1^2 + w_2^2 - w_3^2 + w_4^2); %Plus Configuration
% tau_psi = (b * w_1^2 + Im) - (b * w_2^2 + Im) + (b * w_3^2 + Im) - (b * w_4^2 + Im);

== matlab function Quadrotor_Model_PID_Control_Updated/Quadrotor Dynamic Model/Subsystem p_dot/MATLAB Function ==
  data: w_2 input; w_4 input; tau_phi output
function tau_phi = fcn(w_2, w_4)
k = 2.980e-6; % Thrust factor of rotor (depends on density
              % geometry, etc) 
l = 0.225; % Linear distance from the centre of the rotor
           % to the centre of gravity          
tau_phi = l * k * (-w_2^2 + w_4^2);

%Eqn 13

== matlab function Quadrotor_Model_PID_Control_Updated/Quadrotor Dynamic Model/Subsystem q_dot/MATLAB Function1 ==
  data: w_1 input; w_3 input; tau_theta output
function tau_theta = fcn(w_1, w_3)
k = 2.980e-6; % Thrust factor of rotor (depends on density
              % geometry, etc) 
l = 0.225; % Linear distance from the centre of the rotor
           % to the centre of gravity          
tau_theta = l * k * (-w_1^2 + w_3^2);

== matlab function Quadrotor_Model_PID_Control_Updated/Quadrotor Dynamic Model/Thrust ==
  data: w_1 input; Thrust output; w_2 input; w_3 input; w_4 input
function Thrust = fcn(w_1, w_2, w_3, w_4)
k = 2.980e-6; % Thrust factor of rotor (depends on density)
Thrust = k * (w_1^2 + w_2^2 + w_3^2 + w_4^2);
